simulink model "verify_RealTimePulse_mdl"  (R2016b)
settings: Solver=FixedStepAuto  StartTime=0  StopTime=5  FixedStep=1  RelTol=1e-3  EnableMultiTasking=on
libraries: carnot x3
settings Model: Creator=drhf  LastModifiedBy=drhf
settings DataIOCC: SaveFormat=Array  SignalLoggingSaveFormat=ModelDataLogs
settings OptimizationCC: ExpressionDepthLimit=2147483647  LifeSpan=inf
settings DebuggingCC: UnderspecifiedInitializationDetection=Classic  MergeDetectMultiDrivingBlocksExec=none  SolverPrmCheckMsg=warning  FcnCallInpInsideContextMsg=warning  StateNameClashWarn=warning  SFUnexpectedBacktrackingDiag=warning  SFNoUnconditionalDefaultTransitionDiag=warning  SFExecutionAtInitializationDiag=none
settings HardwareCC: ProdBitPerPointer=32  ProdBitPerSizeT=32  ProdBitPerPtrDiffT=32  ProdLargestAtomicFloat=None  ProdIntDivRoundTo=Undefined  ProdEndianess=Unspecified  ProdWordSize=32  ProdHWDeviceType=32-bit Generic
settings ModelReferenceCC: PropagateSignalLabelsOutOfModel=off
settings GRTTargetCC: TargetLangStandard=C89/C90 (ANSI)  GeneratePreprocessorConditionals=Disable all  CombineOutputUpdateFcns=off  GRTInterface=on
settings ConfigComp: CovMetricSettings=dw  CovHtmlReporting=on  CovSaveCumulativeToWorkspaceVar=on  CovSaveSingleToWorkspaceVar=on  CovExternalEMLEnable=off

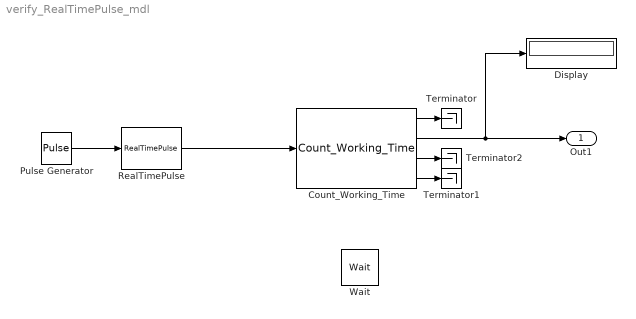
== system verify_RealTimePulse_mdl ==
  Count_Working_Time : carnot/Toolbox/Count_Working_Time
  Display : Display
  Pulse Generator : DiscretePulseGenerator  PulseType=Time based  PulseWidth=50  PhaseDelay=1
  RealTimePulse : carnot/Toolbox/RealTimePulse  typ=rising  time=1
  Terminator : Terminator
  Terminator1 : Terminator
  Terminator2 : Terminator
  Wait : carnot/Toolbox/Wait  check=off  date=[1 10 15 31 00]  wtime=1
  Out1 : Outport
  wires:
  RealTimePulse/1 -> Count_Working_Time/1
  Pulse Generator/1 -> RealTimePulse/1
  Count_Working_Time/1 -> Terminator/1
  Count_Working_Time/3 -> Terminator2/1
  Count_Working_Time/2 -> Display/1, Out1/1
  Count_Working_Time/4 -> Terminator1/1
